simulink model "vector_reference"  (Simulink 6.3)
settings: Solver=ode45  StartTime=0.0  StopTime=6179  RelTol=1e-3
undefined symbols (not defined in the file): drag_coef, ff_on, I_sat, omega_init, q_init, R_ref_E, ro_air
libraries: components_lib x43, simulink x9
settings Model: Creator=krage  LastModifiedBy=mnkr02  ExtModeAutoUpdateStatusClock=off  StrictBusMsg=None

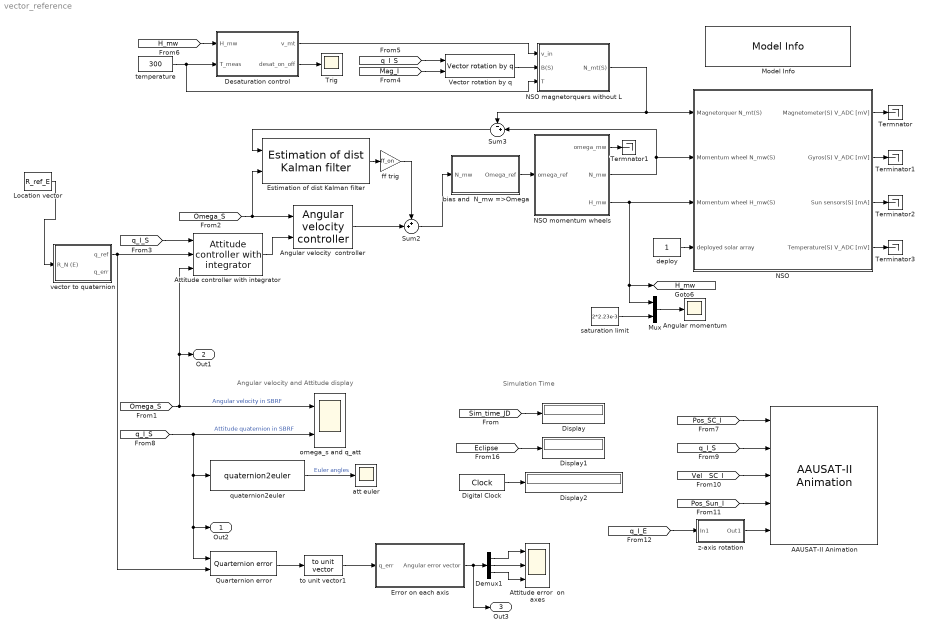
== system vector_reference ==
  note: Simulation Time
  note: Angular velocity and Attitude display
  AAUSAT-II Animation : components_lib/Other model utilities/AAUSAT-II Animation  u1=[-20000000 20000000 -20000000 20000000 -20000000 20000000]  u2=50  u3=500000  u20=on  u18=15  u4=6.371e6  u11=150  u12=on  u13='earth2150.jpg'  u17=180  u5=Fixed position  u6=[-20000000 -9000000 70000000]  u7=12  u9=on  u10=off  u16=off  u14=on  u15=on  u8=on  u19=on
  Angular momentum : Scope
      settings: YMin=0.00125  YMax=0.0045  SaveName=ScopeData2
  Angular velocity  controller : components_lib/ACS/Controllers/Angular velocity  controller  ang_file_name='ang_robust_control.m'
  Attitude controller with integrator : components_lib/ACS/Controllers/Attitude controller with integrator  att_file_name='att_control_with_integrator.m'
  Attitude error  on axes : Scope  NumInputPorts=3
      settings: YMin=0.25~0~0.5  YMax=2.25~1~2.25  SaveName=ScopeData5
  Demux1 : Demux  Outputs=3
  Desaturation control : Subsystem  mask{h_bias=2.23*1e-3, desat_on=0.7*2.23e-3, desat_off=0.01*2.23e-3}
      mask prompts: h_bias "Angular momentum bias"; desat_on "Threshold desaturation on"; desat_off "Threshold desaturation off"
  Digital Clock : DigitalClock
  Display : Display
  Display1 : Display
  Display2 : Display
  Error on each axis : Subsystem
  Estimation of dist Kalman filter : components_lib/ACS/Controllers/Estimation of dist Kalman filter  ang_file_name='kalman_estimator.m'
  Location vector : Constant  Value=R_ref_E
  Model Info : simulink/Model-Wide Utilities/Model Info  InitialBlockCM=None  BlockCM=None  Frame=on  DisplayStringWithTags=|  HorizontalTextAlignment=Center  LeftAlignmentValue=0.5  SourceBlockDiagram=vector_reference  TagMaxNumber=20
      | sun to eclipse : 2452315.560376
      | 32 sec. before : 2452315.56
      | eclipse to sun : 2452315.513363
  Mux : Mux  Inputs=2
  NSO : Subsystem  Tag=AAUSAT-II Model  Description=AAUSAT-II Model  AncestorBlock=components_lib/NSO  mask{r_com_s=[0.05 0.05 0.15], sat_temp_start=0, r_com_s_deployed=[0.05 0.05 0.125], mass_sc=3, Dim=[0.1 0.1 0.3], inertia_c=[25 25 5]/1e3, inertia_d=I_sat, init_jd=2452315.56, q_s_c=[0 0 0 1], q_init_s_i=q_init, w_init_s=omega_init, Cd=drag_coef, rho=ro_air, enable_sensor_emulation=off, alb_emu_enabled=off, enable_dist=on}
      mask prompts: r_com_s "Center of mass (S)"; sat_temp_start "Start temperature of satellite [K]"; r_com_s_deployed "Center of mass (deployed)"; mass_sc "Mass of spacecraft (kg)"; Dim "Dimensions of the satellite (m)"; inertia_c "Folded inertia matrix(C)"; inertia_d "Deployed inertia matrix(C)"; init_jd "Initial time (JD)"; q_s_c "Controller reference frame (S->C)"; q_init_s_i "Initial attitude q_i(S->I)"; w_init_s "Initial angular rate W(S)"; Cd "Drag Coefficient"; rho "Air Density"; enable_sensor_emulation "Enable sensor emulation?"; alb_emu_enabled "Enable albedo emulation?"; enable_dist "Enable disturbances"
      mask Display:
      | image(imread('NSO.jpg'));
      | color('r');
      | port_label('input', 1, 'N_mt(S)');
      | port_label('input', 2, 'N_mw(S)');
      | port_label('input', 3, 'H_mw(S)');
      | port_label('input', 4, 'Deployed solar array');
      | port_label('output', 1, 'Magnetometer(S) V_ADC [mV]');
      | port_label('output', 2, 'Gyros(S) V_ADC [mV]');
      | port_label('output', 3, 'Sun sensors(S) [mA]');
      | port_label('output', 4, 'Temperature(S) V_ADC [mV]');
  NSO magnetorquers without L : Subsystem  AncestorBlock=components_lib/Actuator Emulation/NSO magnetorquers without L
  NSO momentum wheels : Subsystem  AncestorBlock=components_lib/Actuator Emulation/NSO momentum wheels  mask{w_mw_i=[1078.6 1078.6 1078.6] *0.5}
      mask prompts: w_mw_i "Initial Angular Velocity"
  Quarternion error : components_lib/Math utilities/Quaternion operations/Quarternion error
  Sum2 : Sum  Inputs=++|
  Sum3 : Sum  Orientation=left  Inputs=-+|
  Terminator1 : Terminator
  Terminator2 : Terminator
  Terminator3 : Terminator
  Termnator : Terminator
  Termnator1 : Terminator
  Trig : Scope
      settings: YMin=0.95  YMax=1.05  SaveName=ScopeData3
  Vector rotation by q : components_lib/Math utilities/Quaternion operations/Vector rotation by q
  att euler : Scope
      settings: YMin=-3.5  YMax=3.5
  bias and  N_mw =>Omega : Subsystem
  deploy : Constant
  ff trig : Gain  Gain=ff_on
  omega_s and q_att : Scope  NumInputPorts=2
      settings: YMin=-0.125~-1  YMax=0.125~1
  quaternion2euler : components_lib/Math utilities/Quaternion operations/quaternion2euler
  saturation limit : Constant  Value=2*2.23e-3
  temperature : Constant  Value=300
  to unit vector1 : components_lib/Math utilities/Vector operations/to unit vector
  vector to quaternion : Subsystem
  z-axis rotation : Subsystem
  Out2 : Outport
  Out1 : Outport  Port=2
  Out3 : Outport  Port=3
  tag scope: H_mw=global
  wires:
  [q_I_S] -> omega_s and q_att/2, quaternion2euler/1, Out2/1, Quarternion error/1  "Attitude quaternion in SBRF"
  quaternion2euler/1 -> att euler/1  "Euler angles"
  [Sim_time_JD] -> Display/1
  [Eclipse] -> Display1/1
  Digital Clock/1 -> Display2/1
  deploy/1 -> NSO/4(deployed solar array)
  [q_I_S] -> Attitude controller with integrator/1
  [Omega_S] -> Angular velocity  controller/1, Estimation of dist Kalman filter/2
  Attitude controller with integrator/1 -> Angular velocity  controller/2
  temperature/1 -> Desaturation control/2(T_meas), NSO magnetorquers without L/3(T)
  [Mag_I] -> Vector rotation by q/2
  [q_I_S] -> Vector rotation by q/1
  Vector rotation by q/1 -> NSO magnetorquers without L/2(B(S))
  Desaturation control/1(v_mt) -> NSO magnetorquers without L/1(v_in)
  [H_mw] -> Desaturation control/1(H_mw)
  NSO magnetorquers without L/1(N_mt(S)) -> NSO/1(Magnetorquer N_mt(S)), Sum3/1
  Desaturation control/2(desat_on_off) -> Trig/1
  NSO momentum wheels/3(H_mw) -> [H_mw], Mux/1, NSO/3(Momentum wheel H_mw(S))
  NSO momentum wheels/2(N_mw) -> Sum3/2, NSO/2(Momentum wheel N_mw(S))
  bias and  N_mw =>Omega/1(Omega_ref) -> NSO momentum wheels/1(omega_ref)
  Mux/1 -> Angular momentum/1
  saturation limit/1 -> Mux/2
  [Omega_S] -> omega_s and q_att/1, Out1/1, Attitude controller with integrator/3  "Angular velocity in SBRF"
  Angular velocity  controller/1 -> Sum2/2
  Sum2/1 -> bias and  N_mw =>Omega/1(N_mw)
  Sum3/1 -> Estimation of dist Kalman filter/1
  NSO/1(Magnetometer(S) V_ADC [mV]) -> Termnator/1
  NSO/2(Gyros(S) V_ADC [mV]) -> Terminator1/1
  NSO/3(Sun sensors(S) [mA]) -> Terminator2/1
  NSO/4(Temperature(S) V_ADC [mV]) -> Terminator3/1
  Estimation of dist Kalman filter/1 -> ff trig/1
  ff trig/1 -> Sum2/1
  Quarternion error/1 -> to unit vector1/1
  Error on each axis/1(Angular error vector) -> Demux1/1, Out3/1
  Demux1/1 -> Attitude error  on axes/1
  Demux1/2 -> Attitude error  on axes/2
  Demux1/3 -> Attitude error  on axes/3
  [q_I_E] -> z-axis rotation/1(In1)
  z-axis rotation/1(Out1) -> AAUSAT-II Animation/5
  [Pos_SC_I] -> AAUSAT-II Animation/1
  [q_I_S] -> AAUSAT-II Animation/2
  [Vel__SC_I] -> AAUSAT-II Animation/3
  [Pos_Sun_I] -> AAUSAT-II Animation/4
  vector to quaternion/1(q_ref) -> Quarternion error/2, Attitude controller with integrator/2
  to unit vector1/1 -> Error on each axis/1(q_err)
  NSO momentum wheels/1(omega_mw) -> Termnator1/1
  Location vector/1 -> vector to quaternion/1(R_N (E))

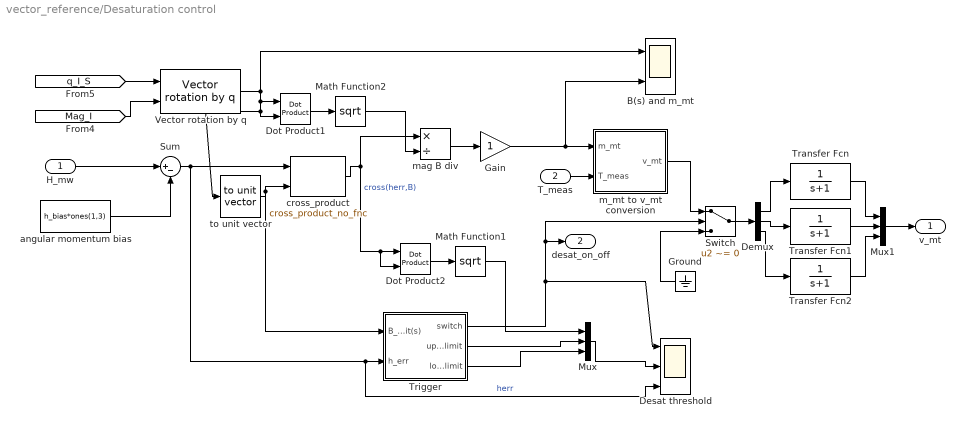
== system vector_reference/Desaturation control ==
  H_mw : Inport
  T_meas : Inport  Port=2
  B(s) and m_mt : Scope  NumInputPorts=2
      settings: YMin=-2e-005~-1  YMax=2e-005~11  SaveName=ScopeData6
  Demux : Demux  Outputs=3
  Desat threshold : Scope  NumInputPorts=3
      settings: YMin=0~0~-0.0025  YMax=1~0.004~0.0025  SaveName=desat_info
  Dot Product1 : simulink/Math Operations/Dot Product  InputSameDT=on  OutDataType=sfix(16)  OutScaling=2^-10  DoSatur=off
  Dot Product2 : simulink/Math Operations/Dot Product  InputSameDT=on  OutDataType=sfix(16)  OutScaling=2^-10  DoSatur=off
  Gain : Gain
  Ground : Ground  Orientation=left
  Math Function1 : Math  Operator=sqrt  SaturateOnIntegerOverflow=on
  Math Function2 : Math  Operator=sqrt  SaturateOnIntegerOverflow=on
  Mux : Mux  Inputs=3
  Mux1 : Mux  Inputs=3
  Sum : Sum  Inputs=|+-
  Switch : Switch  Criteria=u2 ~= 0  Threshold=0.5
  Transfer Fcn : TransferFcn  Denominator=[1 1]
  Transfer Fcn1 : TransferFcn  Denominator=[1 1]
  Transfer Fcn2 : TransferFcn  Denominator=[1 1]
  Trigger : Subsystem
  Vector rotation by q : components_lib/Math utilities/Quaternion operations/Vector rotation by q
  angular momentum bias : Constant  Value=h_bias*ones(1,3)
  cross_product : components_lib/Math utilities/Vector operations/cross_product_no_fnc
  m_mt to v_mt conversion : Subsystem  mask{n_mt=[435 435 865], A_mt=[0.21*0.07 0.21*0.07 0.07*0.07], L_mt=[26.956e-3 26.956e-3 59.256e-3], v_max_mt=5}
      mask prompts: n_mt "Coil winding number [n_x n_y n_z]"; A_mt "Coil area [A_mt_x A_mt_y A_mt_z]"; L_mt "Coil inductance [L_mt_x L_mt_y L_mt_z]"; v_max_mt "Maximum voltage"
  mag B div : Product  Inputs=*/  OutScaling=2^-10
  to unit vector : components_lib/Math utilities/Vector operations/to unit vector
  v_mt : Outport
  desat_on_off : Outport  Port=2
  wires:
  H_mw/1 -> Sum/1
  angular momentum bias/1 -> Sum/2
  [Mag_I] -> Vector rotation by q/2
  [q_I_S] -> Vector rotation by q/1
  Sum/1 -> cross_product/1, Trigger/2(h_err), Desat threshold/3  "herr"
  Vector rotation by q/1 -> Dot Product1/1, Dot Product1/2, to unit vector/1, B(s) and m_mt/1
  cross_product/1 -> mag B div/1, Dot Product2/1, Dot Product2/2  "cross(herr,B)"
  Ground/1 -> Switch/3
  T_meas/1 -> m_mt to v_mt conversion/2(T_meas)
  mag B div/1 -> Gain/1
  m_mt to v_mt conversion/1(v_mt) -> Switch/1
  Dot Product1/1 -> Math Function2/1
  Math Function2/1 -> mag B div/2
  Gain/1 -> m_mt to v_mt conversion/1(m_mt), B(s) and m_mt/2
  to unit vector/1 -> cross_product/2, Trigger/1(B_unit(s))
  Switch/1 -> Demux/1
  Demux/1 -> Transfer Fcn/1
  Demux/2 -> Transfer Fcn1/1
  Demux/3 -> Transfer Fcn2/1
  Transfer Fcn/1 -> Mux1/1
  Transfer Fcn1/1 -> Mux1/2
  Transfer Fcn2/1 -> Mux1/3
  Mux1/1 -> v_mt/1
  Mux/1 -> Desat threshold/2
  Trigger/1(switch) -> Desat threshold/1, desat_on_off/1, Switch/2
  Trigger/2(upper limit) -> Mux/2
  Dot Product2/1 -> Math Function1/1
  Math Function1/1 -> Mux/1
  Trigger/3(lower limit) -> Mux/3

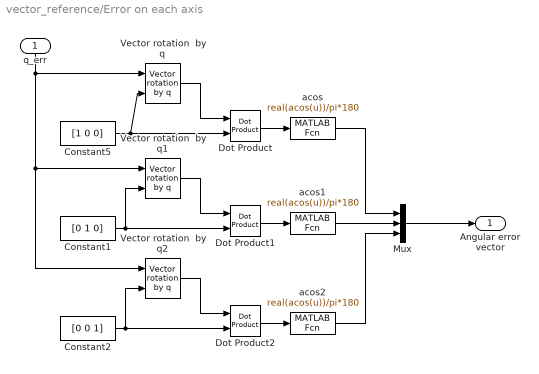
== system vector_reference/Error on each axis ==
  q_err : Inport  Orientation=down
  Constant1 : Constant  Value=[0 1 0]
  Constant2 : Constant  Value=[0 0 1]
  Constant5 : Constant  Value=[1 0 0]
  Dot Product : simulink/Math Operations/Dot Product  InputSameDT=on  OutDataType=sfix(16)  OutScaling=2^-10  DoSatur=off
  Dot Product1 : simulink/Math Operations/Dot Product  InputSameDT=on  OutDataType=sfix(16)  OutScaling=2^-10  DoSatur=off
  Dot Product2 : simulink/Math Operations/Dot Product  InputSameDT=on  OutDataType=sfix(16)  OutScaling=2^-10  DoSatur=off
  Mux : Mux  Inputs=3
  Vector rotation  by q : components_lib/Math utilities/Quaternion operations/Vector rotation by q
  Vector rotation  by q1 : components_lib/Math utilities/Quaternion operations/Vector rotation by q
  Vector rotation  by q2 : components_lib/Math utilities/Quaternion operations/Vector rotation by q
  acos : MATLABFcn  MATLABFcn=real(acos(u))/pi*180
  acos1 : MATLABFcn  MATLABFcn=real(acos(u))/pi*180
  acos2 : MATLABFcn  MATLABFcn=real(acos(u))/pi*180
  Angular error vector : Outport
  wires:
  Constant5/1 -> Dot Product/2, Vector rotation  by q/2
  Vector rotation  by q/1 -> Dot Product/1
  Dot Product/1 -> acos/1
  q_err/1 -> Vector rotation  by q/1, Vector rotation  by q1/1, Vector rotation  by q2/1
  Constant1/1 -> Vector rotation  by q1/2, Dot Product1/2
  Vector rotation  by q1/1 -> Dot Product1/1
  Dot Product1/1 -> acos1/1
  Constant2/1 -> Vector rotation  by q2/2, Dot Product2/2
  Vector rotation  by q2/1 -> Dot Product2/1
  Dot Product2/1 -> acos2/1
  acos/1 -> Mux/1
  acos1/1 -> Mux/2
  acos2/1 -> Mux/3
  Mux/1 -> Angular error vector/1

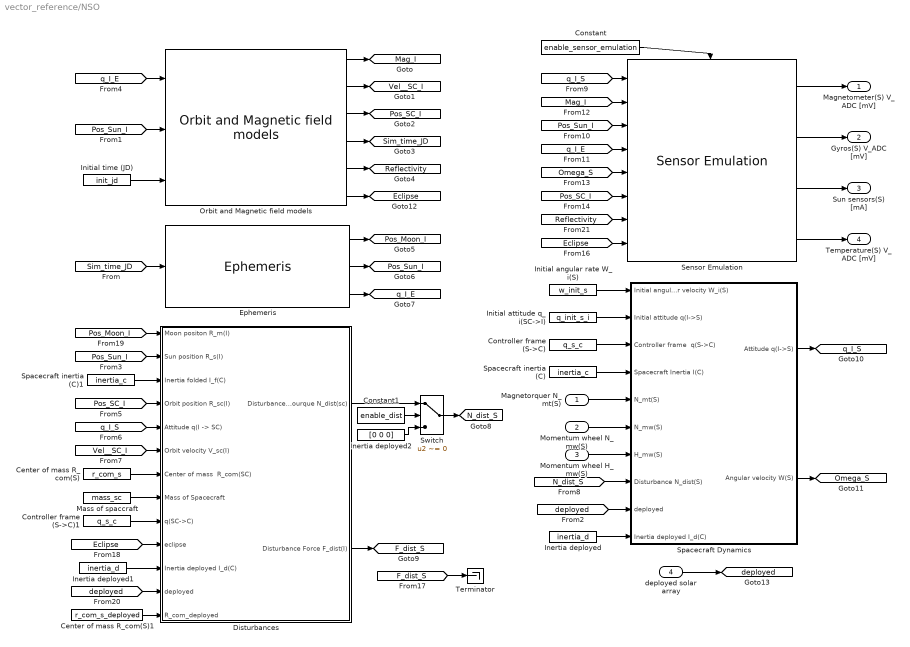
== system vector_reference/NSO ==
  Magnetorquer N_mt(S) : Inport
  Momentum wheel N_mw(S) : Inport  Port=2
  Momentum wheel H_mw(S) : Inport  Port=3
  deployed solar array : Inport  Port=4
  Center of mass R_com(S) : Constant  Value=r_com_s
  Center of mass R_com(S)1 : Constant  Value=r_com_s_deployed
  Constant : Constant  Value=enable_sensor_emulation
  Constant1 : Constant  Value=enable_dist
  Controller frame (S->C) : Constant  Value=q_s_c
  Controller frame (S->C)1 : Constant  Value=q_s_c
  Disturbances : Subsystem  AncestorBlock=components_lib/Disturbances/Disturbances
  Ephemeris : components_lib/Orbit and Ephemeris/Ephemeris
  Inertia deployed : Constant  Value=inertia_d
  Inertia deployed1 : Constant  Value=inertia_d
  Inertia deployed2 : Constant  Value=[0 0 0]
  Initial angular rate W_i(S) : Constant  Value=w_init_s
  Initial attitude q_i(SC->I) : Constant  Value=q_init_s_i
  Initial time (JD) : Constant  Value=init_jd
  Mass of spaccraft : Constant  Value=mass_sc
  Orbit and Magnetic field models : components_lib/Orbit and Ephemeris/Orbit and Magnetic field models  data_type=SGP4/IGRF models  tle_type=Oersted TLE  reflectivity_enabled=0
  Sensor Emulation : components_lib/Sensor Emulation/Sensor Emulation
  Spacecraft Dynamics : Subsystem  AncestorBlock=components_lib/Dynamics and Kinematics/Spacecraft Dynamics
  Spacecraft inertia (C) : Constant  Value=inertia_c
  Spacecraft inertia (C)1 : Constant  Value=inertia_c
  Switch : Switch  Criteria=u2 ~= 0
  Terminator : Terminator
  Magnetometer(S) V_ADC [mV] : Outport
  Gyros(S) V_ADC [mV] : Outport  Port=2
  Sun sensors(S) [mA] : Outport  Port=3
  Temperature(S) V_ADC [mV] : Outport  Port=4
  tag scope: Eclipse=global, F_dist_S=global, Mag_I=global, N_dist_S=global, Omega_S=global, Pos_Moon_I=global, Pos_SC_I=global, Pos_Sun_I=global, Reflectivity=global, Sim_time_JD=global, Vel__SC_I=global, deployed=global, q_I_E=global, q_I_S=global
  wires:
  Inertia deployed1/1 -> Disturbances/11(Inertia deployed I_d(C))
  [deployed] -> Disturbances/12(deployed)
  [deployed] -> Spacecraft Dynamics/9(deployed)
  Inertia deployed/1 -> Spacecraft Dynamics/10(Inertia deployed I_d(C))
  deployed solar array/1 -> [deployed]
  [F_dist_S] -> Terminator/1
  [Eclipse] -> Sensor Emulation/8
  Orbit and Magnetic field models/6 -> [Eclipse]
  Sensor Emulation/4 -> Temperature(S) V_ADC [mV]/1
  Magnetorquer N_mt(S)/1 -> Spacecraft Dynamics/5(N_mt(S))
  Momentum wheel H_mw(S)/1 -> Spacecraft Dynamics/7(H_mw(S))
  Controller frame (S->C)1/1 -> Disturbances/9(q(SC->C))
  Mass of spaccraft/1 -> Disturbances/8("Mass of Spacecraft ")
  Orbit and Magnetic field models/1 -> [Mag_I]
  Sensor Emulation/1 -> Magnetometer(S) V_ADC [mV]/1
  Sensor Emulation/2 -> Gyros(S) V_ADC [mV]/1
  Sensor Emulation/3 -> Sun sensors(S) [mA]/1
  Orbit and Magnetic field models/2 -> [Vel__SC_I]
  [q_I_E] -> Orbit and Magnetic field models/1
  Center of mass R_com(S)/1 -> Disturbances/7(Center of mass  R_com(SC))
  Spacecraft inertia (C)1/1 -> Disturbances/3(Inertia folded I_f(C))
  Spacecraft inertia (C)/1 -> Spacecraft Dynamics/4(Spacecraft Inertia I(C))
  Controller frame (S->C)/1 -> Spacecraft Dynamics/3(Controller frame  q(S->C))
  Orbit and Magnetic field models/3 -> [Pos_SC_I]
  Initial angular rate W_i(S)/1 -> Spacecraft Dynamics/1(Initial angular velocity W_i(S))
  Initial attitude q_i(SC->I)/1 -> Spacecraft Dynamics/2(Initial attitude q(I->S))
  Orbit and Magnetic field models/4 -> [Sim_time_JD]
  Ephemeris/1 -> [Pos_Moon_I]
  Ephemeris/2 -> [Pos_Sun_I]
  Ephemeris/3 -> [q_I_E]
  Orbit and Magnetic field models/5 -> [Reflectivity]
  Disturbances/2(Disturbance Force F_dist(I)) -> [F_dist_S]
  Spacecraft Dynamics/1(Attitude q(I->S)) -> [q_I_S]
  Spacecraft Dynamics/2(Angular velocity W(S)) -> [Omega_S]
  [Sim_time_JD] -> Ephemeris/1
  [Pos_Sun_I] -> Orbit and Magnetic field models/2
  [Pos_Moon_I] -> Disturbances/1(Moon positon R_m(I))
  [Pos_Sun_I] -> Disturbances/2(Sun position R_s(I))
  Initial time (JD)/1 -> Orbit and Magnetic field models/3
  [Pos_SC_I] -> Disturbances/4(Orbit position R_sc(I))
  [q_I_S] -> Disturbances/5("Attitude q(I -> SC)")
  [Vel__SC_I] -> Disturbances/6(Orbit velocity V_sc(I))
  [q_I_S] -> Sensor Emulation/1
  [Pos_Sun_I] -> Sensor Emulation/3
  [Mag_I] -> Sensor Emulation/2
  [q_I_E] -> Sensor Emulation/4
  [Omega_S] -> Sensor Emulation/5
  [Pos_SC_I] -> Sensor Emulation/6
  [Reflectivity] -> Sensor Emulation/7
  [Eclipse] -> Disturbances/10(eclipse)
  Momentum wheel N_mw(S)/1 -> Spacecraft Dynamics/6(N_mw(S))
  Center of mass R_com(S)1/1 -> Disturbances/13(R_com_deployed)
  [N_dist_S] -> Spacecraft Dynamics/8(Disturbance N_dist(S))
  Disturbances/1(Disturbance tourque N_dist(sc)) -> Switch/1
  Constant/1 -> Sensor Emulation/Enable
  Constant1/1 -> Switch/2
  Inertia deployed2/1 -> Switch/3
  Switch/1 -> [N_dist_S]

== system vector_reference/NSO magnetorquers without L ==
  v_in : Inport
  B(S) : Inport  Port=2
  T : Inport  Port=3
  Add : Sum  Inputs=+++  OutScaling=2^-10
  Add1 : Sum  Inputs=+++  OutScaling=2^-10
  Demux : Demux  Outputs=3
  Integrator : Integrator
  Scope : Scope
      settings: YMin=24.35  YMax=25.2  SaveName=power_mt
  "X Magnetorquer  without L " : Subsystem  AncestorBlock=components_lib/Actuator Emulation/Magnetorquer without L  mask{v_max_mt=5, coil_dim=[0.07 0.21], n_mt=435, A_wire_mt=(pi/4)*0.0002^2, sigma_0_mt=1.7e-8, alpha_0_mt=3.9e-3, T_0_mt=293}
      mask prompts: v_max_mt "Maximum voltage"; coil_dim "Coil dimensions [x y]"; n_mt "Coil winding number"; A_wire_mt "Wire cross sectional area"; sigma_0_mt "Wire resistivity"; alpha_0_mt "Wire resistivity temp. coef."; T_0_mt "Wire resistivity base temp."
  X coil  normal : Constant  Value=[1;0;0]
  Y Magnetorquer  without L : Subsystem  AncestorBlock=components_lib/Actuator Emulation/Magnetorquer without L  mask{v_max_mt=5, coil_dim=[0.07 0.21], n_mt=435, A_wire_mt=(pi/4)*0.0002^2, sigma_0_mt=1.7e-8, alpha_0_mt=3.9e-3, T_0_mt=293}
      mask prompts: v_max_mt "Maximum voltage"; coil_dim "Coil dimensions [x y]"; n_mt "Coil winding number"; A_wire_mt "Wire cross sectional area"; sigma_0_mt "Wire resistivity"; alpha_0_mt "Wire resistivity temp. coef."; T_0_mt "Wire resistivity base temp."
  Y coil normal : Constant  Value=[0;1;0]
  Z Magnetorquer  without L : Subsystem  AncestorBlock=components_lib/Actuator Emulation/Magnetorquer without L  mask{v_max_mt=5, coil_dim=[0.07 0.07], n_mt=865, A_wire_mt=(pi/4)*0.0002^2, sigma_0_mt=1.7e-8, alpha_0_mt=3.9e-3, T_0_mt=293}
      mask prompts: v_max_mt "Maximum voltage"; coil_dim "Coil dimensions [x y]"; n_mt "Coil winding number"; A_wire_mt "Wire cross sectional area"; sigma_0_mt "Wire resistivity"; alpha_0_mt "Wire resistivity temp. coef."; T_0_mt "Wire resistivity base temp."
  Z coil normal : Constant  Value=[0;0;1]
  N_mt(S) : Outport  PortDimensions=3
  wires:
  v_in/1 -> Demux/1
  Add/1 -> N_mt(S)/1
  X coil  normal/1 -> "X Magnetorquer  without L "/2(coil normal)
  Demux/1 -> "X Magnetorquer  without L "/1(v_mt)
  "X Magnetorquer  without L "/1(N_mt(s)) -> Add/1
  Y Magnetorquer  without L/1(N_mt(s)) -> Add/2
  Z Magnetorquer  without L/1(N_mt(s)) -> Add/3
  Demux/2 -> Y Magnetorquer  without L/1(v_mt)
  Y coil normal/1 -> Y Magnetorquer  without L/2(coil normal)
  Demux/3 -> Z Magnetorquer  without L/1(v_mt)
  Z coil normal/1 -> Z Magnetorquer  without L/2(coil normal)
  B(S)/1 -> Z Magnetorquer  without L/3(B(s)), Y Magnetorquer  without L/3(B(s)), "X Magnetorquer  without L "/3(B(s))
  T/1 -> Z Magnetorquer  without L/4(T), Y Magnetorquer  without L/4(T), "X Magnetorquer  without L "/4(T)
  "X Magnetorquer  without L "/2(P_mt) -> Add1/1
  Y Magnetorquer  without L/2(P_mt) -> Add1/2
  Z Magnetorquer  without L/2(P_mt) -> Add1/3
  Add1/1 -> Integrator/1
  Integrator/1 -> Scope/1

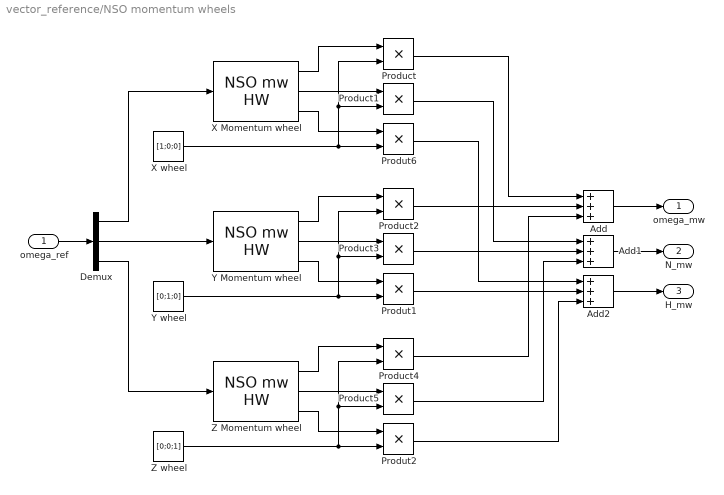
== system vector_reference/NSO momentum wheels ==
  omega_ref : Inport
  Add : Sum  Inputs=+++  OutScaling=2^-10
  Add1 : Sum  Inputs=+++  OutScaling=2^-10
  Add2 : Sum  Inputs=+++  OutScaling=2^-10
  Demux : Demux  Outputs=3
  Product{,1..5} (6 alike) : Product  RndMeth=Zero
  Produt1 : Product  RndMeth=Zero
  Produt2 : Product  RndMeth=Zero
  Produt6 : Product  RndMeth=Zero
  X Momentum wheel : components_lib/Actuator Emulation/NSO mw HW  C_p=0.01  C_i=0.001  w_mw_init=w_mw_i(1)
  X wheel : Constant  Value=[1;0;0]
  Y Momentum wheel : components_lib/Actuator Emulation/NSO mw HW  C_p=0.01  C_i=0.001  w_mw_init=w_mw_i(2)
  Y wheel : Constant  Value=[0;1;0]
  Z Momentum wheel : components_lib/Actuator Emulation/NSO mw HW  C_p=0.01  C_i=0.001  w_mw_init=w_mw_i(3)
  Z wheel : Constant  Value=[0;0;1]
  omega_mw : Outport  PortDimensions=3
  N_mw : Outport  Port=2  PortDimensions=3
  H_mw : Outport  Port=3  PortDimensions=3
  wires:
  Demux/2 -> Y Momentum wheel/1
  Demux/3 -> Z Momentum wheel/1
  Demux/1 -> X Momentum wheel/1
  omega_ref/1 -> Demux/1
  Product4/1 -> Add/3
  Product5/1 -> Add1/3
  Produt2/1 -> Add2/3
  Z Momentum wheel/2 -> Product5/1
  Z Momentum wheel/1 -> Product4/1
  Z Momentum wheel/3 -> Produt2/1
  Z wheel/1 -> Produt2/2, Product5/2, Product4/2
  Produt1/1 -> Add2/2
  Product3/1 -> Add1/2
  Product2/1 -> Add/2
  Y Momentum wheel/2 -> Product3/1
  Y Momentum wheel/1 -> Product2/1
  Y Momentum wheel/3 -> Produt1/1
  Y wheel/1 -> Produt1/2, Product3/2, Product2/2
  X Momentum wheel/2 -> Product1/1
  X Momentum wheel/1 -> Product/1
  X Momentum wheel/3 -> Produt6/1
  Add/1 -> omega_mw/1
  X wheel/1 -> Produt6/2, Product1/2, Product/2
  Add1/1 -> N_mw/1
  Product/1 -> Add/1
  Product1/1 -> Add1/1
  Add2/1 -> H_mw/1
  Produt6/1 -> Add2/1

== system vector_reference/bias and  N_mw =>Omega ==
  N_mw : Inport
  I_FW : Gain  Gain=1/4.139e-6
  Integrator : Integrator
  Sum : Sum  Inputs=|++
  angular velocity bias : Constant  Value=[1078.6 1078.6 1078.6] *0.5
  Omega_ref : Outport
  wires:
  I_FW/1 -> Sum/1
  angular velocity bias/1 -> Sum/2
  Integrator/1 -> I_FW/1
  N_mw/1 -> Integrator/1
  Sum/1 -> Omega_ref/1

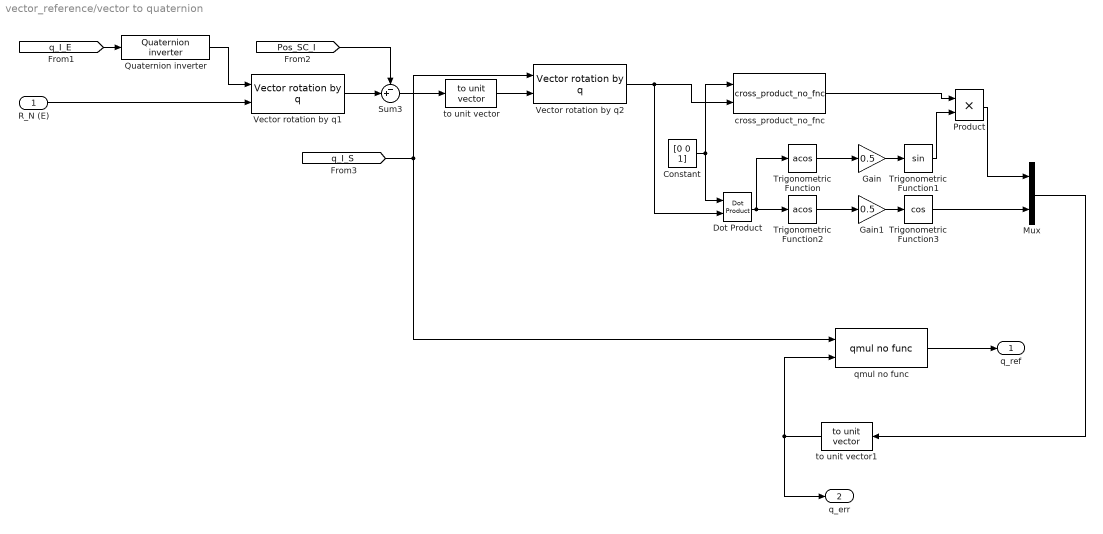
== system vector_reference/vector to quaternion ==
  R_N (E) : Inport
  Constant : Constant  Value=[0 0 1]
  Dot Product : simulink/Math Operations/Dot Product  InputSameDT=on  OutDataType=sfix(16)  OutScaling=2^-10  DoSatur=off
  Gain : Gain  Gain=0.5
  Gain1 : Gain  Gain=0.5
  Mux : Mux  Inputs=2
  Product : Product  RndMeth=Zero
  Quaternion inverter : components_lib/Math utilities/Quaternion operations/Quaternion inverter
  Sum3 : Sum  Inputs=-+|
  Trigonometric Function : Trigonometry  Operator=acos
  Trigonometric Function1 : Trigonometry
  Trigonometric Function2 : Trigonometry  Operator=acos
  Trigonometric Function3 : Trigonometry  Operator=cos
  Vector rotation by q1 : components_lib/Math utilities/Quaternion operations/Vector rotation by q
  Vector rotation by q2 : components_lib/Math utilities/Quaternion operations/Vector rotation by q
  cross_product_no_fnc : components_lib/Math utilities/Vector operations/cross_product_no_fnc
  qmul no func : components_lib/Math utilities/Quaternion operations/qmul no func
  to unit vector : components_lib/Math utilities/Vector operations/to unit vector
  to unit vector1 : components_lib/Math utilities/Vector operations/to unit vector  Orientation=left
  q_ref : Outport
  q_err : Outport  Port=2
  wires:
  [q_I_E] -> Quaternion inverter/1
  R_N (E)/1 -> Vector rotation by q1/2
  Vector rotation by q1/1 -> Sum3/2
  [Pos_SC_I] -> Sum3/1
  Quaternion inverter/1 -> Vector rotation by q1/1
  [q_I_S] -> Vector rotation by q2/1, qmul no func/1
  Sum3/1 -> to unit vector/1
  Vector rotation by q2/1 -> Dot Product/2, cross_product_no_fnc/2
  Constant/1 -> Dot Product/1, cross_product_no_fnc/1
  Dot Product/1 -> Trigonometric Function/1, Trigonometric Function2/1
  Trigonometric Function/1 -> Gain/1
  cross_product_no_fnc/1 -> Product/1
  Trigonometric Function1/1 -> Product/2
  Product/1 -> Mux/1
  Mux/1 -> to unit vector1/1
  qmul no func/1 -> q_ref/1
  Gain/1 -> Trigonometric Function1/1
  Trigonometric Function2/1 -> Gain1/1
  Gain1/1 -> Trigonometric Function3/1
  Trigonometric Function3/1 -> Mux/2
  to unit vector/1 -> Vector rotation by q2/2
  to unit vector1/1 -> qmul no func/2, q_err/1

== system vector_reference/z-axis rotation ==
  In1 : Inport
  Demux2 : Demux
  Gain : Gain  Gain=2
  Subsystem : Subsystem
  Trigonometric Function : Trigonometry  Operator=acos
  Out1 : Outport
  wires:
  Demux2/4 -> Trigonometric Function/1
  Trigonometric Function/1 -> Gain/1
  Demux2/1 -> Subsystem/1(In1)
  Demux2/2 -> Subsystem/2(In2)
  Demux2/3 -> Subsystem/3(In3)
  In1/1 -> Demux2/1
  Gain/1 -> Out1/1

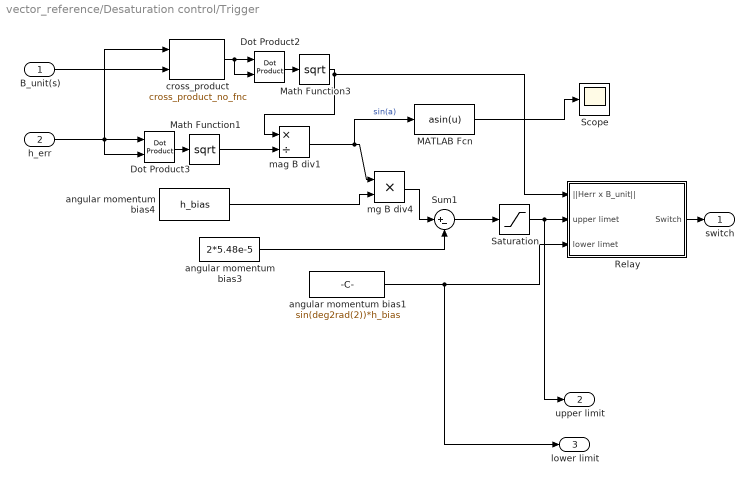
== system vector_reference/Desaturation control/Trigger ==
  B_unit(s) : Inport  PortDimensions=3
  h_err : Inport  Port=2
  Dot Product2 : simulink/Math Operations/Dot Product  InputSameDT=on  OutDataType=sfix(16)  OutScaling=2^-10  DoSatur=off
  Dot Product3 : simulink/Math Operations/Dot Product  InputSameDT=on  OutDataType=sfix(16)  OutScaling=2^-10  DoSatur=off
  MATLAB Fcn : MATLABFcn  MATLABFcn=asin(u)
  Math Function1 : Math  Operator=sqrt  SaturateOnIntegerOverflow=on
  Math Function3 : Math  Operator=sqrt  SaturateOnIntegerOverflow=on
  Relay : Subsystem
  Saturation : Saturate  UpperLimit=inf  LowerLimit=2*sin(deg2rad(2))*h_bias
  Scope : Scope
      settings: YMin=0.5  YMax=1.6  SaveName=ScopeData4
  Sum1 : Sum  Inputs=|+-
  angular momentum bias1 : Constant  Value=sin(deg2rad(2))*h_bias
  angular momentum bias3 : Constant  Value=2*5.48e-5
  angular momentum bias4 : Constant  Value=h_bias
  cross_product : components_lib/Math utilities/Vector operations/cross_product_no_fnc
  mag B div1 : Product  Inputs=*/  OutScaling=2^-10
  mg B div4 : Product  OutScaling=2^-10
  switch : Outport
  upper limit : Outport  Port=2
  lower limit : Outport  Port=3
  wires:
  angular momentum bias3/1 -> Sum1/2
  Relay/1(Switch) -> switch/1
  angular momentum bias4/1 -> mg B div4/2
  mg B div4/1 -> Sum1/1
  Dot Product2/1 -> Math Function3/1
  Dot Product3/1 -> Math Function1/1
  Math Function1/1 -> mag B div1/2
  Sum1/1 -> Saturation/1
  mag B div1/1 -> mg B div4/1, MATLAB Fcn/1  "sin(a)"
  h_err/1 -> Dot Product3/1, Dot Product3/2, cross_product/1
  B_unit(s)/1 -> cross_product/2
  cross_product/1 -> Dot Product2/1, Dot Product2/2
  Math Function3/1 -> mag B div1/1, Relay/1(||Herr x B_unit||)
  angular momentum bias1/1 -> Relay/3(lower limet), lower limit/1
  MATLAB Fcn/1 -> Scope/1
  Saturation/1 -> Relay/2(upper limet), upper limit/1

== system vector_reference/Desaturation control/m_mt to v_mt conversion ==
  m_mt : Inport
  T_meas : Inport  Port=2
  Demux : Demux  Outputs=3
  Gain : Gain  Gain=1/(n_mt(1)*A_mt(1))
  Gain1 : Gain  Gain=1/(n_mt(2)*A_mt(2))
  Gain2 : Gain  Gain=1/(n_mt(3)*A_mt(3))
  Mux : Mux  Inputs=3
  Resistance for mt on x-axis : Subsystem  mask{A_wire_mt=(pi/4)*0.0002^2, sigma_0_mt=1.7e-8, alpha_0_mt=3.9e-3, T_0_mt=293}
      mask prompts: A_wire_mt "Wire cross sectional area"; sigma_0_mt "Wire resistivity"; alpha_0_mt "Wire resistivity temp. coef."; T_0_mt "Wire resistivity base temp."
  Resistance for mt on y-axis : Subsystem  mask{A_wire_mt=(pi/4)*0.0002^2, sigma_0_mt=1.7e-8, alpha_0_mt=3.9e-3, T_0_mt=293}
      mask prompts: A_wire_mt "Wire cross sectional area"; sigma_0_mt "Wire resistivity"; alpha_0_mt "Wire resistivity temp. coef."; T_0_mt "Wire resistivity base temp."
  Resistance for mt on z-axis : Subsystem  mask{A_wire_mt=(pi/4)*0.0002^2, sigma_0_mt=1.7e-8, alpha_0_mt=3.9e-3, T_0_mt=293}
      mask prompts: A_wire_mt "Wire cross sectional area"; sigma_0_mt "Wire resistivity"; alpha_0_mt "Wire resistivity temp. coef."; T_0_mt "Wire resistivity base temp."
  electromechanis transfer funtion for mt_x : Subsystem
  "electromechanis transfer funtion for mt_y " : Subsystem
  "electromechanis transfer funtion for mt_z " : Subsystem
  i_mt : Scope  NumInputPorts=3
      settings: YMin=-5~-5~-5  YMax=5~5~5  SaveName=ScopeData8
  v_mt : Outport
  wires:
  Demux/3 -> Gain2/1
  Demux/2 -> Gain1/1
  Demux/1 -> Gain/1
  Gain/1 -> electromechanis transfer funtion for mt_x/1(i_mt), i_mt/1
  Gain1/1 -> "electromechanis transfer funtion for mt_y "/1(i_mt), i_mt/2
  Gain2/1 -> "electromechanis transfer funtion for mt_z "/1(i_mt), i_mt/3
  m_mt/1 -> Demux/1
  "electromechanis transfer funtion for mt_y "/1(v_mt) -> Mux/2
  "electromechanis transfer funtion for mt_z "/1(v_mt) -> Mux/3
  Resistance for mt on x-axis/1(R(T)) -> electromechanis transfer funtion for mt_x/2(R(T))
  Resistance for mt on y-axis/1(R(T)) -> "electromechanis transfer funtion for mt_y "/2(R(T))
  Resistance for mt on z-axis/1(R(T)) -> "electromechanis transfer funtion for mt_z "/2(R(T))
  T_meas/1 -> Resistance for mt on y-axis/1(T), Resistance for mt on x-axis/1(T), Resistance for mt on z-axis/1(T)
  electromechanis transfer funtion for mt_x/1(v_mt) -> Mux/1
  Mux/1 -> v_mt/1

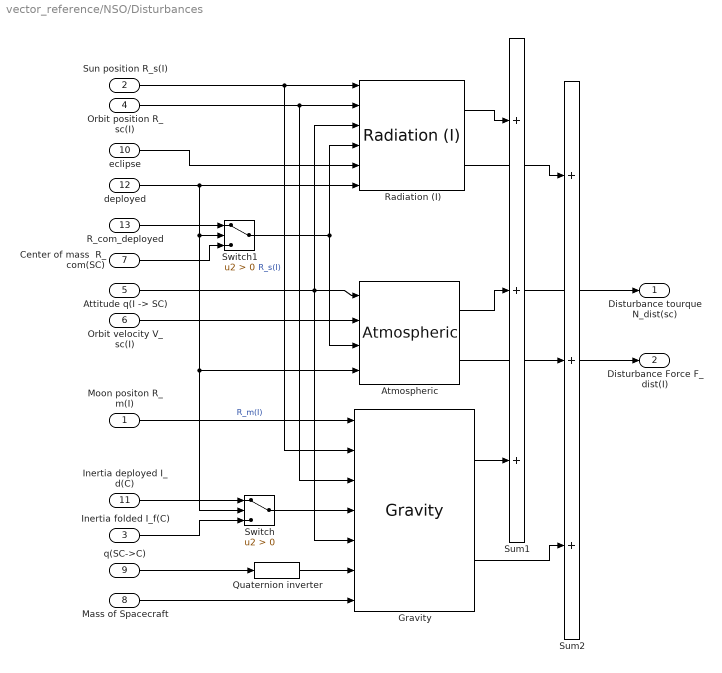
== system vector_reference/NSO/Disturbances ==
  Moon positon R_m(I) : Inport
  Sun position R_s(I) : Inport  Port=2
  Inertia folded I_f(C) : Inport  Port=3
  Orbit position R_sc(I) : Inport  Port=4
  "Attitude q(I -> SC)" : Inport  Port=5
  Orbit velocity V_sc(I) : Inport  Port=6
  Center of mass  R_com(SC) : Inport  Port=7
  "Mass of Spacecraft " : Inport  Port=8
  q(SC->C) : Inport  Port=9
  eclipse : Inport  Port=10
  Inertia deployed I_d(C) : Inport  Port=11
  deployed : Inport  Port=12
  R_com_deployed : Inport  Port=13
  Atmospheric : components_lib/Disturbances/Atmospheric
  Gravity : components_lib/Disturbances/Gravity  G=6.673e-11  M_sun=1.98892e30  M_moon=7.36e22  M_earth=5.9742e24
  Quaternion inverter : components_lib/Math utilities/Quaternion operations/Quaternion inverter
  Radiation (I) : components_lib/Disturbances/Radiation (I)
  Sum1 : Sum  Inputs=+++  SaturateOnIntegerOverflow=on
  Sum2 : Sum  Inputs=+++  SaturateOnIntegerOverflow=on
  Switch : Switch  Criteria=u2 > Threshold
  Switch1 : Switch  Criteria=u2 > Threshold
  Disturbance tourque N_dist(sc) : Outport
  Disturbance Force F_dist(I) : Outport  Port=2
  wires:
  Switch1/1 -> Atmospheric/3, Radiation (I)/4
  R_com_deployed/1 -> Switch1/1
  Center of mass  R_com(SC)/1 -> Switch1/3
  q(SC->C)/1 -> Quaternion inverter/1
  Quaternion inverter/1 -> Gravity/6
  "Mass of Spacecraft "/1 -> Gravity/7
  Moon positon R_m(I)/1 -> Gravity/1  "R_m(I)"
  Sun position R_s(I)/1 -> Gravity/2, Radiation (I)/1  "R_s(I)"
  "Attitude q(I -> SC)"/1 -> Atmospheric/1, Radiation (I)/3, Gravity/5
  Orbit position R_sc(I)/1 -> Gravity/3, Radiation (I)/2
  Orbit velocity V_sc(I)/1 -> Atmospheric/2
  Radiation (I)/1 -> Sum1/1
  Atmospheric/1 -> Sum1/2
  Gravity/1 -> Sum1/3
  Radiation (I)/2 -> Sum2/1
  Atmospheric/2 -> Sum2/2
  Gravity/2 -> Sum2/3
  Sum1/1 -> Disturbance tourque N_dist(sc)/1
  Sum2/1 -> Disturbance Force F_dist(I)/1
  eclipse/1 -> Radiation (I)/5
  Inertia folded I_f(C)/1 -> Switch/3
  Inertia deployed I_d(C)/1 -> Switch/1
  Switch/1 -> Gravity/4
  deployed/1 -> Switch1/2, Switch/2, Atmospheric/4, Radiation (I)/6

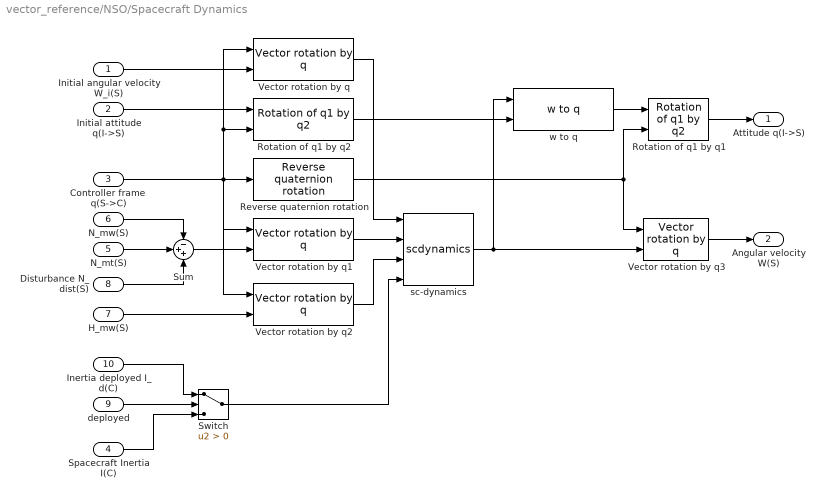
== system vector_reference/NSO/Spacecraft Dynamics ==
  Initial angular velocity W_i(S) : Inport
  Initial attitude q(I->S) : Inport  Port=2
  Controller frame  q(S->C) : Inport  Port=3
  Spacecraft Inertia I(C) : Inport  Port=4
  N_mt(S) : Inport  Port=5
  N_mw(S) : Inport  Port=6
  H_mw(S) : Inport  Port=7
  Disturbance N_dist(S) : Inport  Port=8
  deployed : Inport  Port=9
  Inertia deployed I_d(C) : Inport  Port=10
  Reverse quaternion rotation : components_lib/Math utilities/Quaternion operations/Reverse quaternion rotation
  Rotation of q1 by q1 : components_lib/Math utilities/Quaternion operations/Rotation of q1 by q2
  Rotation of q1 by q2 : components_lib/Math utilities/Quaternion operations/Rotation of q1 by q2
  Sum : Sum  Inputs=-++  SaturateOnIntegerOverflow=on
  Switch : Switch  Criteria=u2 > Threshold
  Vector rotation by q{,1..3} (4 alike) : components_lib/Math utilities/Vector operations/Vector rotation by q
  sc-dynamics : S-Function  FunctionName=scdynamics
  w to q : components_lib/Math utilities/Quaternion operations/w to q
  Attitude q(I->S) : Outport
  Angular velocity W(S) : Outport  Port=2
  wires:
  deployed/1 -> Switch/2
  Spacecraft Inertia I(C)/1 -> Switch/3
  Inertia deployed I_d(C)/1 -> Switch/1
  Switch/1 -> sc-dynamics/4
  Sum/1 -> Vector rotation by q1/2
  Initial angular velocity W_i(S)/1 -> Vector rotation by q/2
  Controller frame  q(S->C)/1 -> Vector rotation by q2/1, Reverse quaternion rotation/1, Vector rotation by q1/1, Rotation of q1 by q2/2, Vector rotation by q/1
  Initial attitude q(I->S)/1 -> Rotation of q1 by q2/1
  Vector rotation by q/1 -> sc-dynamics/1
  Vector rotation by q2/1 -> sc-dynamics/3
  Reverse quaternion rotation/1 -> Rotation of q1 by q1/2, Vector rotation by q3/1
  Vector rotation by q3/1 -> Angular velocity W(S)/1
  Rotation of q1 by q2/1 -> w to q/2
  w to q/1 -> Rotation of q1 by q1/1
  H_mw(S)/1 -> Vector rotation by q2/2
  sc-dynamics/1 -> w to q/1, Vector rotation by q3/2
  Rotation of q1 by q1/1 -> Attitude q(I->S)/1
  Vector rotation by q1/1 -> sc-dynamics/2
  N_mt(S)/1 -> Sum/2
  Disturbance N_dist(S)/1 -> Sum/3
  N_mw(S)/1 -> Sum/1

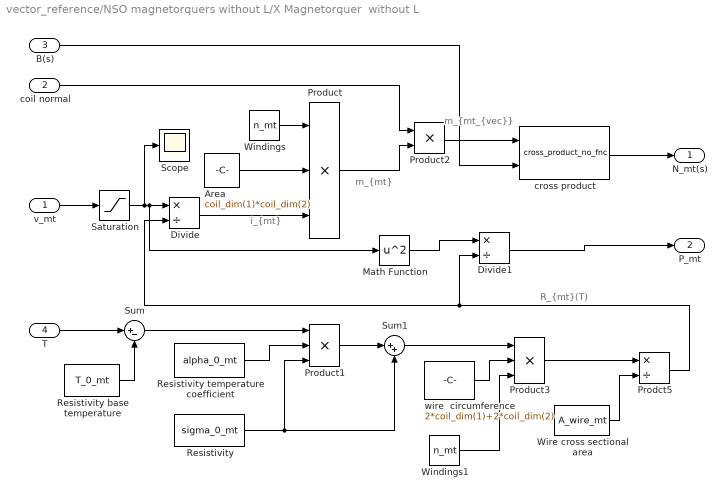
== system vector_reference/NSO magnetorquers without L/X Magnetorquer  without L  ==
  note: R_{mt}(T)
  note: i_{mt}
  note: m_{mt}
  note: m_{mt_{vec}}
  v_mt : Inport
  coil normal : Inport  Port=2
  B(s) : Inport  Port=3
  T : Inport  Port=4
  Area : Constant  Value=coil_dim(1)*coil_dim(2)
  Divide : Product  Inputs=*/  OutScaling=2^-10
  Divide1 : Product  Inputs=*/  OutScaling=2^-10
  Math Function : Math  Operator=square  SaturateOnIntegerOverflow=on
  Prodct5 : Product  Inputs=*/  RndMeth=Zero
  Product : Product  Inputs=3  RndMeth=Zero
  Product1 : Product  Inputs=3  RndMeth=Zero
  Product2 : Product  RndMeth=Zero
  Product3 : Product  Inputs=3  RndMeth=Zero
  Resistivity : Constant  Value=sigma_0_mt
  Resistivity base temperature : Constant  Value=T_0_mt
  Resistivity temperature coefficient : Constant  Value=alpha_0_mt
  Saturation : Saturate  UpperLimit=v_max_mt  LowerLimit=-v_max_mt
  Scope : Scope
      settings: SaveName=ScopeData12
  Sum : Sum  Inputs=|+-
  Sum1 : Sum  Inputs=|++
  Windings : Constant  Value=n_mt
  Windings1 : Constant  Value=n_mt
  Wire cross sectional area : Constant  Value=A_wire_mt
  cross product : components_lib/Math utilities/Vector operations/cross_product_no_fnc
  wire  circumference : Constant  Value=2*coil_dim(1)+2*coil_dim(2)
  N_mt(s) : Outport
  P_mt : Outport  Port=2
  wires:
  Prodct5/1 -> Divide/2, Divide1/2
  Wire cross sectional area/1 -> Prodct5/2
  Product3/1 -> Prodct5/1
  Windings1/1 -> Product3/3
  wire  circumference/1 -> Product3/2
  Sum1/1 -> Product3/1
  Product1/1 -> Sum1/1
  Resistivity/1 -> Sum1/2, Product1/3
  Sum/1 -> Product1/1
  Resistivity temperature coefficient/1 -> Product1/2
  T/1 -> Sum/1
  Resistivity base temperature/1 -> Sum/2
  coil normal/1 -> Product2/1
  v_mt/1 -> Saturation/1
  Saturation/1 -> Divide/1, Math Function/1, Scope/1
  Divide/1 -> Product/3
  Windings/1 -> Product/1
  Area/1 -> Product/2
  Product/1 -> Product2/2
  Product2/1 -> cross product/1
  cross product/1 -> N_mt(s)/1
  B(s)/1 -> cross product/2
  Math Function/1 -> Divide1/1
  Divide1/1 -> P_mt/1

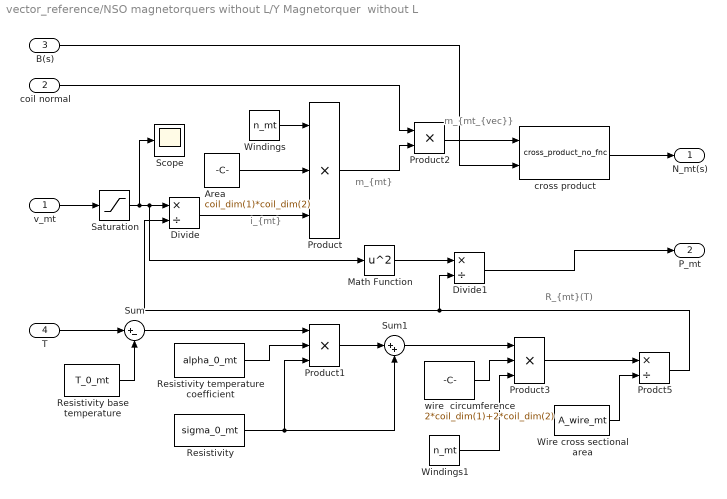
== system vector_reference/NSO magnetorquers without L/Y Magnetorquer  without L ==
  note: R_{mt}(T)
  note: i_{mt}
  note: m_{mt}
  note: m_{mt_{vec}}
  v_mt : Inport
  coil normal : Inport  Port=2
  B(s) : Inport  Port=3
  T : Inport  Port=4
  Area : Constant  Value=coil_dim(1)*coil_dim(2)
  Divide : Product  Inputs=*/  OutScaling=2^-10
  Divide1 : Product  Inputs=*/  OutScaling=2^-10
  Math Function : Math  Operator=square  SaturateOnIntegerOverflow=on
  Prodct5 : Product  Inputs=*/  RndMeth=Zero
  Product : Product  Inputs=3  RndMeth=Zero
  Product1 : Product  Inputs=3  RndMeth=Zero
  Product2 : Product  RndMeth=Zero
  Product3 : Product  Inputs=3  RndMeth=Zero
  Resistivity : Constant  Value=sigma_0_mt
  Resistivity base temperature : Constant  Value=T_0_mt
  Resistivity temperature coefficient : Constant  Value=alpha_0_mt
  Saturation : Saturate  UpperLimit=v_max_mt  LowerLimit=-v_max_mt
  Scope : Scope
      settings: SaveName=ScopeData13
  Sum : Sum  Inputs=|+-
  Sum1 : Sum  Inputs=|++
  Windings : Constant  Value=n_mt
  Windings1 : Constant  Value=n_mt
  Wire cross sectional area : Constant  Value=A_wire_mt
  cross product : components_lib/Math utilities/Vector operations/cross_product_no_fnc
  wire  circumference : Constant  Value=2*coil_dim(1)+2*coil_dim(2)
  N_mt(s) : Outport
  P_mt : Outport  Port=2
  wires:
  Prodct5/1 -> Divide/2, Divide1/2
  Wire cross sectional area/1 -> Prodct5/2
  Product3/1 -> Prodct5/1
  Windings1/1 -> Product3/3
  wire  circumference/1 -> Product3/2
  Sum1/1 -> Product3/1
  Product1/1 -> Sum1/1
  Resistivity/1 -> Sum1/2, Product1/3
  Sum/1 -> Product1/1
  Resistivity temperature coefficient/1 -> Product1/2
  T/1 -> Sum/1
  Resistivity base temperature/1 -> Sum/2
  coil normal/1 -> Product2/1
  v_mt/1 -> Saturation/1
  Saturation/1 -> Divide/1, Math Function/1, Scope/1
  Divide/1 -> Product/3
  Windings/1 -> Product/1
  Area/1 -> Product/2
  Product/1 -> Product2/2
  Product2/1 -> cross product/1
  cross product/1 -> N_mt(s)/1
  B(s)/1 -> cross product/2
  Math Function/1 -> Divide1/1
  Divide1/1 -> P_mt/1

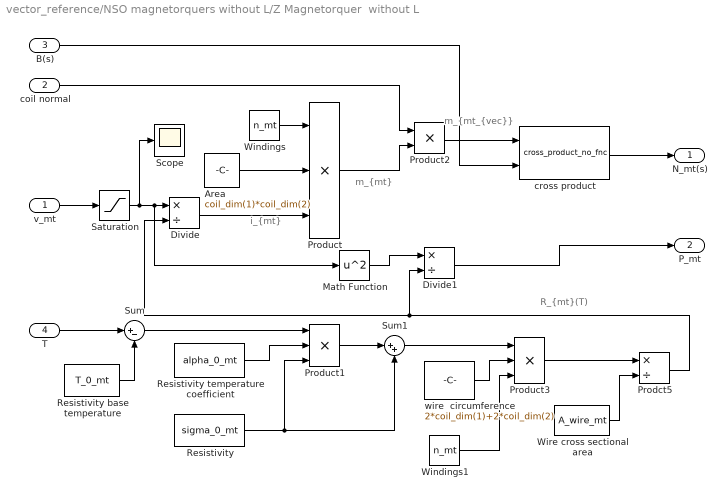
== system vector_reference/NSO magnetorquers without L/Z Magnetorquer  without L ==
  note: R_{mt}(T)
  note: i_{mt}
  note: m_{mt}
  note: m_{mt_{vec}}
  v_mt : Inport
  coil normal : Inport  Port=2
  B(s) : Inport  Port=3
  T : Inport  Port=4
  Area : Constant  Value=coil_dim(1)*coil_dim(2)
  Divide : Product  Inputs=*/  OutScaling=2^-10
  Divide1 : Product  Inputs=*/  OutScaling=2^-10
  Math Function : Math  Operator=square  SaturateOnIntegerOverflow=on
  Prodct5 : Product  Inputs=*/  RndMeth=Zero
  Product : Product  Inputs=3  RndMeth=Zero
  Product1 : Product  Inputs=3  RndMeth=Zero
  Product2 : Product  RndMeth=Zero
  Product3 : Product  Inputs=3  RndMeth=Zero
  Resistivity : Constant  Value=sigma_0_mt
  Resistivity base temperature : Constant  Value=T_0_mt
  Resistivity temperature coefficient : Constant  Value=alpha_0_mt
  Saturation : Saturate  UpperLimit=v_max_mt  LowerLimit=-v_max_mt
  Scope : Scope
      settings: YMin=-1.5  SaveName=ScopeData14
  Sum : Sum  Inputs=|+-
  Sum1 : Sum  Inputs=|++
  Windings : Constant  Value=n_mt
  Windings1 : Constant  Value=n_mt
  Wire cross sectional area : Constant  Value=A_wire_mt
  cross product : components_lib/Math utilities/Vector operations/cross_product_no_fnc
  wire  circumference : Constant  Value=2*coil_dim(1)+2*coil_dim(2)
  N_mt(s) : Outport
  P_mt : Outport  Port=2
  wires:
  Prodct5/1 -> Divide/2, Divide1/2
  Wire cross sectional area/1 -> Prodct5/2
  Product3/1 -> Prodct5/1
  Windings1/1 -> Product3/3
  wire  circumference/1 -> Product3/2
  Sum1/1 -> Product3/1
  Product1/1 -> Sum1/1
  Resistivity/1 -> Sum1/2, Product1/3
  Sum/1 -> Product1/1
  Resistivity temperature coefficient/1 -> Product1/2
  T/1 -> Sum/1
  Resistivity base temperature/1 -> Sum/2
  coil normal/1 -> Product2/1
  v_mt/1 -> Saturation/1
  Saturation/1 -> Divide/1, Math Function/1, Scope/1
  Divide/1 -> Product/3
  Windings/1 -> Product/1
  Area/1 -> Product/2
  Product/1 -> Product2/2
  Product2/1 -> cross product/1
  cross product/1 -> N_mt(s)/1
  B(s)/1 -> cross product/2
  Math Function/1 -> Divide1/1
  Divide1/1 -> P_mt/1

== system vector_reference/z-axis rotation/Subsystem ==
  In1 : Inport
  In2 : Inport  Port=2
  In3 : Inport  Port=3
  Terminator4 : Terminator
  Terminator5 : Terminator
  Terminator6 : Terminator
  wires:
  In1/1 -> Terminator6/1
  In2/1 -> Terminator4/1
  In3/1 -> Terminator5/1

== system vector_reference/Desaturation control/Trigger/Relay ==
  ||Herr x B_unit|| : Inport  Orientation=down
  upper limet : Inport  Port=2
  lower limet : Inport  Port=3
  Logical Operator1 : Logic  AllPortsSameDT=off  OutDataTypeMode=Boolean
  Logical Operator2 : Logic  Operator=OR  AllPortsSameDT=off  OutDataTypeMode=Boolean
  Logical Operator3 : Logic  AllPortsSameDT=off  OutDataTypeMode=Boolean
  Memory : Memory  Orientation=left
  Relational Operator : RelationalOperator  Operator=>  LogicOutDataTypeMode=Boolean  LogicDataType=1
  Relational Operator1 : RelationalOperator  Operator=>  LogicOutDataTypeMode=Boolean  LogicDataType=1
  Switch : Outport
  wires:
  ||Herr x B_unit||/1 -> Relational Operator/1, Relational Operator1/1
  Relational Operator1/1 -> Logical Operator1/1, Logical Operator3/2
  Logical Operator1/1 -> Logical Operator2/2
  Logical Operator2/1 -> Memory/1, Switch/1
  Memory/1 -> Logical Operator1/2
  upper limet/1 -> Relational Operator/2
  lower limet/1 -> Relational Operator1/2
  Relational Operator/1 -> Logical Operator3/1
  Logical Operator3/1 -> Logical Operator2/1

== system vector_reference/Desaturation control/m_mt to v_mt conversion/Resistance for mt on x-axis ==
  T : Inport
  Prodct5 : Product  Inputs=*/  RndMeth=Zero
  Product1 : Product  Inputs=3  RndMeth=Zero
  Product3 : Product  Inputs=3  RndMeth=Zero
  Resistivity : Constant  Value=sigma_0_mt
  Resistivity base temperature : Constant  Value=T_0_mt
  Resistivity temperature coefficient : Constant  Value=alpha_0_mt
  Sum1 : Sum  Inputs=|+-
  Sum2 : Sum  Inputs=|++
  Windings1 : Constant  Value=n_mt(1)
  Wire cross sectional area : Constant  Value=A_wire_mt
  wire  circumference : Constant  Value=4*sqrt(A_mt(1))
  R(T) : Outport
  wires:
  Resistivity base temperature/1 -> Sum1/2
  Resistivity temperature coefficient/1 -> Product1/2
  Sum1/1 -> Product1/1
  Resistivity/1 -> Product1/3, Sum2/2
  Product1/1 -> Sum2/1
  Sum2/1 -> Product3/1
  wire  circumference/1 -> Product3/2
  Windings1/1 -> Product3/3
  Product3/1 -> Prodct5/1
  Wire cross sectional area/1 -> Prodct5/2
  T/1 -> Sum1/1
  Prodct5/1 -> R(T)/1

== system vector_reference/Desaturation control/m_mt to v_mt conversion/Resistance for mt on y-axis ==
  T : Inport
  Prodct5 : Product  Inputs=*/  RndMeth=Zero
  Product1 : Product  Inputs=3  RndMeth=Zero
  Product3 : Product  Inputs=3  RndMeth=Zero
  Resistivity : Constant  Value=sigma_0_mt
  Resistivity base temperature : Constant  Value=T_0_mt
  Resistivity temperature coefficient : Constant  Value=alpha_0_mt
  Sum1 : Sum  Inputs=|+-
  Sum2 : Sum  Inputs=|++
  Windings1 : Constant  Value=n_mt(2)
  Wire cross sectional area : Constant  Value=A_wire_mt
  wire  circumference : Constant  Value=4*sqrt(A_mt(2))
  R(T) : Outport
  wires:
  Prodct5/1 -> R(T)/1
  T/1 -> Sum1/1
  Wire cross sectional area/1 -> Prodct5/2
  Product3/1 -> Prodct5/1
  Windings1/1 -> Product3/3
  wire  circumference/1 -> Product3/2
  Sum2/1 -> Product3/1
  Product1/1 -> Sum2/1
  Resistivity/1 -> Sum2/2, Product1/3
  Sum1/1 -> Product1/1
  Resistivity temperature coefficient/1 -> Product1/2
  Resistivity base temperature/1 -> Sum1/2

== system vector_reference/Desaturation control/m_mt to v_mt conversion/Resistance for mt on z-axis ==
  T : Inport
  Prodct5 : Product  Inputs=*/  RndMeth=Zero
  Product1 : Product  Inputs=3  RndMeth=Zero
  Product3 : Product  Inputs=3  RndMeth=Zero
  Resistivity : Constant  Value=sigma_0_mt
  Resistivity base temperature : Constant  Value=T_0_mt
  Resistivity temperature coefficient : Constant  Value=alpha_0_mt
  Sum1 : Sum  Inputs=|+-
  Sum2 : Sum  Inputs=|++
  Windings1 : Constant  Value=n_mt(3)
  Wire cross sectional area : Constant  Value=A_wire_mt
  wire  circumference : Constant  Value=4*sqrt(A_mt(3))
  R(T) : Outport
  wires:
  Resistivity base temperature/1 -> Sum1/2
  Resistivity temperature coefficient/1 -> Product1/2
  Sum1/1 -> Product1/1
  Resistivity/1 -> Product1/3, Sum2/2
  Product1/1 -> Sum2/1
  Sum2/1 -> Product3/1
  wire  circumference/1 -> Product3/2
  Windings1/1 -> Product3/3
  Product3/1 -> Prodct5/1
  Wire cross sectional area/1 -> Prodct5/2
  T/1 -> Sum1/1
  Prodct5/1 -> R(T)/1

== system vector_reference/Desaturation control/m_mt to v_mt conversion/electromechanis transfer funtion for mt_x ==
  i_mt : Inport
  R(T) : Inport  Port=2
  Derivative : Derivative
  Gain : Gain  Gain=L_mt(1)
  Product1 : Product  RndMeth=Zero
  Scope : Scope  NumInputPorts=3
      settings: YMin=-5~-5~-5  YMax=5~5~5  SaveName=ScopeData9
  Sum : Sum  Inputs=++|
  v_mt : Outport
  wires:
  Derivative/1 -> Gain/1, Scope/1
  Sum/1 -> v_mt/1, Scope/3
  i_mt/1 -> Derivative/1, Product1/1
  R(T)/1 -> Product1/2, Scope/2
  Product1/1 -> Sum/2
  Gain/1 -> Sum/1

== system vector_reference/Desaturation control/m_mt to v_mt conversion/electromechanis transfer funtion for mt_y  ==
  i_mt : Inport
  R(T) : Inport  Port=2
  Derivative : Derivative
  Gain : Gain  Gain=L_mt(2)
  Product1 : Product  RndMeth=Zero
  Sum : Sum  Inputs=++|
  v_mt : Outport
  wires:
  Gain/1 -> Sum/1
  Product1/1 -> Sum/2
  R(T)/1 -> Product1/2
  i_mt/1 -> Product1/1, Derivative/1
  Sum/1 -> v_mt/1
  Derivative/1 -> Gain/1

== system vector_reference/Desaturation control/m_mt to v_mt conversion/electromechanis transfer funtion for mt_z  ==
  i_mt : Inport
  R(T) : Inport  Port=2
  Derivative : Derivative
  Gain : Gain  Gain=L_mt(3)
  Product1 : Product  RndMeth=Zero
  Sum : Sum  Inputs=++|
  v_mt : Outport
  wires:
  Derivative/1 -> Gain/1
  Sum/1 -> v_mt/1
  i_mt/1 -> Derivative/1, Product1/1
  R(T)/1 -> Product1/2
  Product1/1 -> Sum/2
  Gain/1 -> Sum/1
